simulink model "pid_model_2015"  (Simulink 8.5)
settings: Solver=ode45  SolverMode=SingleTasking  StartTime=0.0  StopTime=100  RelTol=1e-3
values from neighbouring files (symbols this model uses):
  G_Denominator = str2double(get(hObject, 'String'))    [gui.m]    (also in variables.mat = [1 -4 3])
  G_Numerator = str2double(get(hObject, 'String'))    [gui.m]    (also in variables.mat = 1)
  H_Denominator = str2double(get(hObject, 'String'))    [gui.m]    (also in variables.mat = 1)
  H_Numerator = str2double(get(hObject, 'String'))    [gui.m]    (also in variables.mat = 1)
  observation_time = 10    [variables.mat]
  PID_D = str2double(get(hObject, 'String'))    [gui.m]    (also in variables.mat = 1000)
  PID_I = str2double(get(hObject, 'String'))    [gui.m]    (also in variables.mat = 0)
  PID_P = str2double(get(hObject, 'String'))    [gui.m]    (also in variables.mat = 17500)
  settling_time = 0.027    [variables.mat]
libraries: simulink x2, vrlib x1
settings Model: Creator=arekmano  LastModifiedBy=Bruce Choi  CovMetricSettings=dwe  CovHtmlReporting=off  covSaveCumulativeToWorkspaceVar=off  CovSaveSingleToWorkspaceVar=off  CovExternalEMLEnable=on
settings DataIOCC: LimitDataPoints=off  SaveFormat=Dataset  SignalLoggingSaveFormat=Dataset
settings OptimizationCC: ExpressionDepthLimit=128
settings DebuggingCC: UnderspecifiedInitializationDetection=Simplified  MergeDetectMultiDrivingBlocksExec=error  FcnCallInpInsideContextMsg=EnableAllAsError  StateNameClashWarn=none  SFUnexpectedBacktrackingDiag=error  SFNoUnconditionalDefaultTransitionDiag=error
settings HardwareCC: ProdBitPerPointer=64  ProdLargestAtomicFloat=Float  ProdIntDivRoundTo=Zero  ProdEndianess=LittleEndian  ProdHWDeviceType=Specified
settings ModelReferenceCC: PropagateSignalLabelsOutOfModel=on
settings GRTTargetCC: TargetLangStandard=C99 (ISO)  GeneratePreprocessorConditionals=Use local settings  CombineOutputUpdateFcns=on  GRTInterface=off

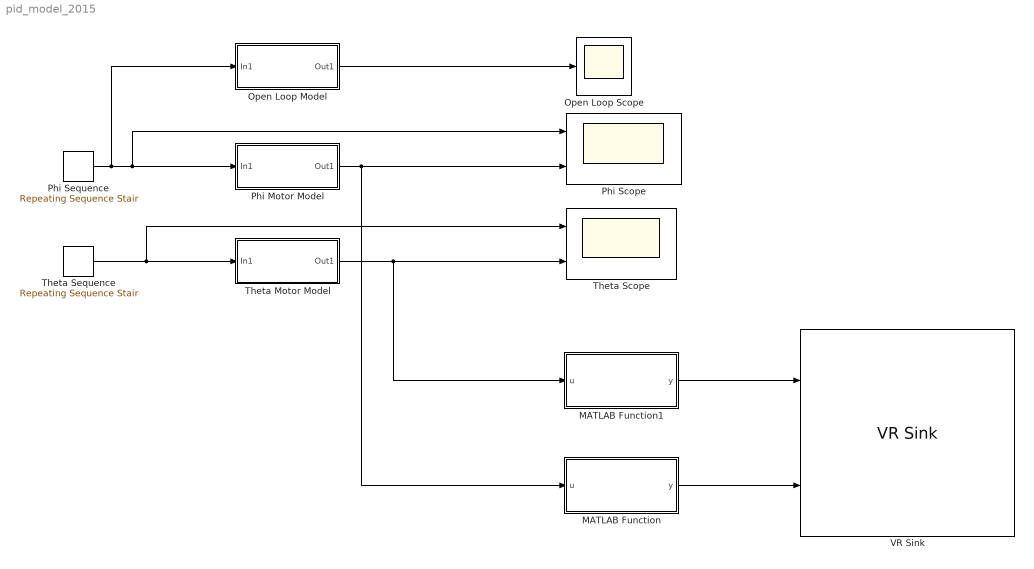
== system pid_model_2015 ==
  MATLAB Function : MATLAB Function  TreatAsAtomicUnit=on
      settings: PermitHierarchicalResolution=ParametersOnly
  MATLAB Function1 : MATLAB Function  TreatAsAtomicUnit=on
      settings: PermitHierarchicalResolution=ParametersOnly
  Open Loop Model : Subsystem
  Open Loop Scope : Scope
      settings: TimeRange=auto  LimitDataPoints=on  MaxDataPoints=5000  SaveToWorkspace=off  SaveName=ScopeData2  YMin=-10  YMax=10  SampleTime=-1  DataFormat=Array
  Phi Motor Model : Subsystem
  Phi Scope : Scope  NumInputPorts=2
      settings: TimeRange=auto  ShowLegends=on  MaxDataPoints=5000  SaveToWorkspace=off  SaveName=ScopeData  YMin=-2.31225~-5  YMax=20.81028~5  SampleTime=-1
  Phi Sequence : simulink/Sources/Repeating Sequence Stair  OutValues=phi_inputs  tsamp=settling_time + observation_time  OutMin=[]  OutMax=[]  OutDataTypeStr=double  OutputDataTypeScalingMode=double  OutDataType=fixdt(0,8)  ConRadixGroup=Best Precision: Vector-wise  OutScaling=2^-12
  Theta Motor Model : Subsystem
  Theta Scope : Scope  NumInputPorts=2
      settings: TimeRange=auto  ShowLegends=on  MaxDataPoints=5000  SaveToWorkspace=off  YMin=-33.39921~-5  YMax=300.59293~5  SampleTime=-1
  Theta Sequence : simulink/Sources/Repeating Sequence Stair  OutValues=theta_inputs  tsamp=settling_time + observation_time  OutMin=[]  OutMax=[]  OutDataTypeStr=double  OutputDataTypeScalingMode=double  OutDataType=fixdt(0,8)  ConRadixGroup=Best Precision: Vector-wise  OutScaling=2^-12
  VR Sink : vrlib/VR Sink  InstantiateOnLoad=on  SampleTime=0.1  ViewEnable=on  RemoteChange=off  RemoteView=off  FieldsWritten=phi.rotation#theta.rotation  WorldFileName=vr_animation.wrl  WorldDescription=The Earth - Low Resolution Model  AutoView=off  VideoDimensions=[]  AllowVariableSize=off  FigureProperties="{'Position', 'Name', 'Viewpoint', 'CameraBound', 'CameraDirection', 'CameraPosition', 'CameraUpVector', 'ZoomFactor', 'Antialiasing', 'Headlight', 'Lighting', 'NavPanel', 'Sound', 'StatusBar', 'Stereo3D', 'Stereo3DCameraOffset', 'Stereo3DHIT', 'ToolBar', 'Textures', 'Transparency', 'Triad', 'Wireframe', 'NavZones', 'NavMode', 'NavSpeed', 'CaptureFileFormat', 'CaptureFileName', 'Record2DCompressMethod', 'Record2DCompressQuality', 'Record2D', 'Record2DFileName', 'Record2DFPS'; [5.0000000000000000e+00   9.2000000000000000e+01   5.7600000000000000e+02   3.5000000000000000e+02], 'The Earth - Low Resolution Model', '', 'on', [0.0000000000000000e+00   0.0000000000000000e+00  -1.0000000000000000e+00], [0.0000000000000000e+00   0.0000000000000000e+00   1.0000000000000000e+01], [0.0000000000000000e+00   1.0000000000000000e+00   0.0000000000000000e+00], [1.0000000000000000e+00], 'on', 'on', 'on', 'halfbar', 'on', 'on', 'off', [1.0000000149011612e-01], [0.0000000000000000e+00], 'on', 'on', 'on', 'none', 'off', 'off', 'fly', 'normal', 'tif', '%f_anim_%n.tif', 'auto', [7.5000000000000000e+01], 'off', '%f_anim_%n.avi', 'auto'}"
  wires:
  Phi Motor Model/1(Out1) -> MATLAB Function/1(u), Phi Scope/2
  Phi Sequence/1 -> Open Loop Model/1(In1), Phi Scope/1, Phi Motor Model/1(In1)
  Theta Sequence/1 -> Theta Scope/1, Theta Motor Model/1(In1)
  Theta Motor Model/1(Out1) -> MATLAB Function1/1(u), Theta Scope/2
  Open Loop Model/1(Out1) -> Open Loop Scope/1
  MATLAB Function1/1(y) -> VR Sink/1
  MATLAB Function/1(y) -> VR Sink/2

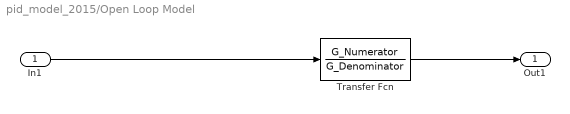
== system pid_model_2015/Open Loop Model ==
  In1 : Inport
  Transfer Fcn : TransferFcn  Numerator=G_Numerator  Denominator=G_Denominator
  Out1 : Outport
  wires:
  Transfer Fcn/1 -> Out1/1
  In1/1 -> Transfer Fcn/1

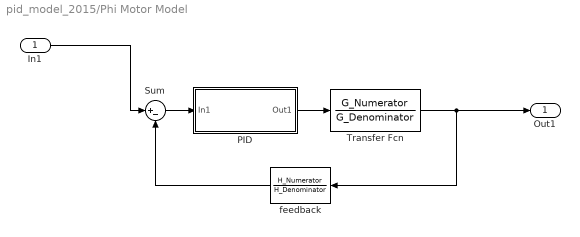
== system pid_model_2015/Phi Motor Model ==
  In1 : Inport
  PID : Subsystem
  Sum : Sum  Inputs=|+-
  Transfer Fcn : TransferFcn  Numerator=G_Numerator  Denominator=G_Denominator
  feedback : TransferFcn  Numerator=H_Numerator  Denominator=H_Denominator
  Out1 : Outport
  wires:
  In1/1 -> Sum/1
  PID/1(Out1) -> Transfer Fcn/1
  Transfer Fcn/1 -> feedback/1, Out1/1
  feedback/1 -> Sum/2
  Sum/1 -> PID/1(In1)

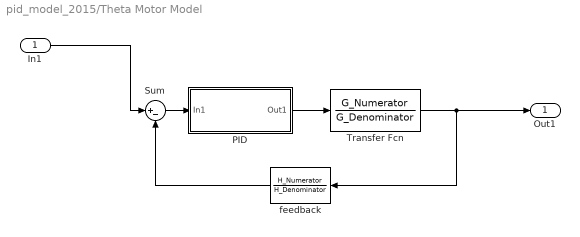
== system pid_model_2015/Theta Motor Model ==
  In1 : Inport
  PID : Subsystem
  Sum : Sum  Inputs=|+-
  Transfer Fcn : TransferFcn  Numerator=G_Numerator  Denominator=G_Denominator
  feedback : TransferFcn  Numerator=H_Numerator  Denominator=H_Denominator
  Out1 : Outport
  wires:
  In1/1 -> Sum/1
  PID/1(Out1) -> Transfer Fcn/1
  Transfer Fcn/1 -> feedback/1, Out1/1
  Sum/1 -> PID/1(In1)
  feedback/1 -> Sum/2

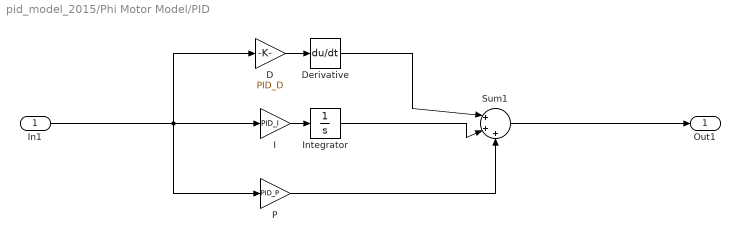
== system pid_model_2015/Phi Motor Model/PID ==
  In1 : Inport
  D : Gain  Gain=PID_D
  Derivative : Derivative
  I : Gain  Gain=PID_I
  Integrator : Integrator
  P : Gain  Gain=PID_P
  Sum1 : Sum  Inputs=|+++
  Out1 : Outport
  wires:
  In1/1 -> P/1, I/1, D/1
  D/1 -> Derivative/1
  I/1 -> Integrator/1
  Integrator/1 -> Sum1/2
  P/1 -> Sum1/3
  Derivative/1 -> Sum1/1
  Sum1/1 -> Out1/1

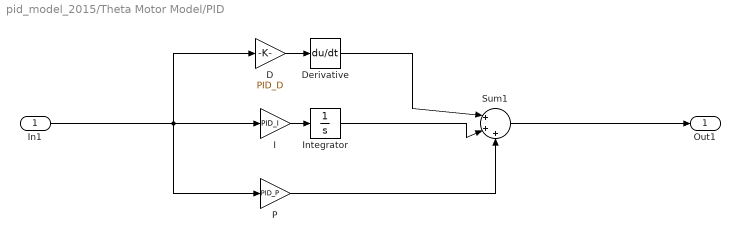
== system pid_model_2015/Theta Motor Model/PID ==
  In1 : Inport
  D : Gain  Gain=PID_D
  Derivative : Derivative
  I : Gain  Gain=PID_I
  Integrator : Integrator
  P : Gain  Gain=PID_P
  Sum1 : Sum  Inputs=|+++
  Out1 : Outport
  wires:
  In1/1 -> P/1, I/1, D/1
  D/1 -> Derivative/1
  I/1 -> Integrator/1
  Integrator/1 -> Sum1/2
  P/1 -> Sum1/3
  Derivative/1 -> Sum1/1
  Sum1/1 -> Out1/1

== matlab function MATLAB Function1 ==
  data: u input double; y output double
function y = fcn(u)

y = [0 1 0 u];

== matlab function MATLAB Function ==
  data: u input double; y output double
function y = fcn(u)

y = [0 0 1 u];
